simulink model "OptFahrzeug1"  (Simulink 5.1)
settings: Solver=ode5  StartTime=0.0  StopTime=max(sim_sample_time)  FixedStep=StepSize  RelTol=1e-3
values from neighbouring files (symbols this model uses):
  drive_acc =     [NoGenDoubleNEDC.mat]
  lm_alternator =     [NoGenDoubleNEDC.mat]
  PwpPt_Tq_EngGross = [0 0 0 1.18647349782e-14 1.38134887733e-14 1.57622425684e-14 1.77109963635e-14 1.96597501586e-14 2.16085039538e-14 2.35572577489e-14 2.5506011544e-14 2.74547653391e-14 ... (23602 elements, 23602x1)]    [NoGenDoubleNEDC.mat]    (also in newdoublecycle.m = [PwpPt_Tq_EngGross;PwpPt_Tq_EngGross])
  PwpPt_W_EngDn = [750 750 750 750 750 750 750 750 750 750 750 750 ... (23602 elements, 23602x1)]    [NoGenDoubleNEDC.mat]    (also in newdoublecycle.m = [PwpPt_W_EngDn;PwpPt_W_EngDn])
  sim_sample_time = [0 0.1 0.2 0.3 0.4 0.5 0.6 0.7 0.8 0.9 1 1.1 ... (23602 elements, 23602x1)]    [NoGenDoubleNEDC.mat]    (also in newdoublecycle.m = [sim_sample_time;sim_sample_time+max(sim_sample_time)+0.1])
  StromTraj = [36.79 ... (first row only)    [StromTrajDef.m]
  ZeitTraj = [0:0.1:-0.1+length(StromTraj)/10]'    [StromTrajDef.m]
settings Model: LastModifiedBy=meifert  ProdHWDeviceType=Microprocessor

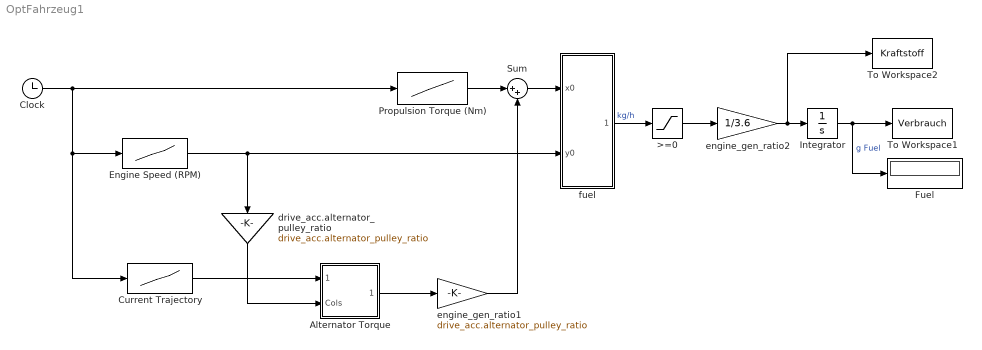
== system OptFahrzeug1 ==
  >=0 : Saturate  UpperLimit=inf  LowerLimit=0
  Alternator Torque : Subsystem  AncestorBlock=|  mask(Lookup Table (2-D)){x=lm_alternator.amp, y=lm_alternator.rpm, t=lm_alternator.loss}
      | simulink3/Functions
      | & Tables/Look-Up
      | Table (2-D)
      mask prompts: x "Row:"; y "Column:"; t "Table:"
      mask help: Performs 2-D linear interpolation of input values using the specified input/output table. Extrapolation is performed outside the table boundaries. The first dimension corresponds to the top (or left) input port.
      mask init:
      | [r,c]=size(t);
      | xt=reshape(x,prod(size(x)),1);
      | xi=xt(:,ones(1,c));
      | minx=min(x); maxx=max(x);
      | mint=min(min(t)); maxt=max(max(t));
      mask Display: plot(double(xi),double(t),double([minx maxx]),double([mint mint]),double([minx minx]),double([mint maxt]))
  Clock : Clock
      settings: Decimation=10
  Current Trajectory : Lookup  InputValues=ZeitTraj  OutputValues=StromTraj  SaturateOnIntegerOverflow=on
  Engine Speed (RPM) : Lookup  InputValues=sim_sample_time  OutputValues=PwpPt_W_EngDn  SaturateOnIntegerOverflow=on
  Fuel : Display
  Integrator : Integrator
  Propulsion Torque (Nm) : Lookup  InputValues=sim_sample_time  OutputValues=PwpPt_Tq_EngGross  SaturateOnIntegerOverflow=on
  Sum : Sum  Inputs=|++  SaturateOnIntegerOverflow=on  InputSameDT=on
  To Workspace1 : ToWorkspace  VariableName=Verbrauch  SampleTime=-1  SaveFormat=Array
  To Workspace2 : ToWorkspace  VariableName=Kraftstoff  SampleTime=-1  SaveFormat=Array
  drive_acc.alternator_pulley_ratio : Gain  Orientation=down  Gain=drive_acc.alternator_pulley_ratio  SaturateOnIntegerOverflow=on
  engine_gen_ratio1 : Gain  Gain=drive_acc.alternator_pulley_ratio  SaturateOnIntegerOverflow=on
  engine_gen_ratio2 : Gain  Gain=1/3.6  SaturateOnIntegerOverflow=on
  fuel : Subsystem  mask(2-D Table Lookup){@1=engine.tq, @2=engine.rpm, @3=engine.fuel}
      mask prompts: @1 "X Index"; @2 "Y Index"; @3 "Table"
      mask help:
      | Two Dimensional Table Lookup
      | The first input corresponds to X Index and the second input corresponds to the Y Index
      mask init:
      | xindex=@1; yindex=@2; table=@3; sftab2chk(xindex,yindex,table);
      mask Help: This block returns a linearly interpolated intersection from the table using the X index (which corresponds to the rows of the table) and the Y index (which corresponds to the columns of the table).  Extrapolation is used.
      mask Display: plot(-10,-10,110,110,[90,50,10],[90,40,30],[90,50,10],[50,26,20],[90,50,10],[22,13,10])
  wires:
  Integrator/1 -> To Workspace1/1, Fuel/1  "g Fuel"
  fuel/1(table out) -> >=0/1  "kg/h"
  >=0/1 -> engine_gen_ratio2/1
  Clock/1 -> Propulsion Torque (Nm)/1, Engine Speed (RPM)/1, Current Trajectory/1
  Engine Speed (RPM)/1 -> drive_acc.alternator_pulley_ratio/1, fuel/2(y0)
  Alternator Torque/1(Out1) -> engine_gen_ratio1/1
  Current Trajectory/1 -> Alternator Torque/1(Rows)
  engine_gen_ratio1/1 -> Sum/2
  Propulsion Torque (Nm)/1 -> Sum/1
  engine_gen_ratio2/1 -> Integrator/1, To Workspace2/1
  drive_acc.alternator_pulley_ratio/1 -> Alternator Torque/2(Cols)
  Sum/1 -> fuel/1(x0)

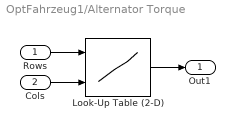
== system OptFahrzeug1/Alternator Torque ==
  Rows : Inport
  Cols : Inport  Port=2
  Look-Up Table (2-D) : Lookup2D  RowIndex=x  ColumnIndex=y  OutputValues=t  SaturateOnIntegerOverflow=on  InputSameDT=on
  Out1 : Outport
  wires:
  Rows/1 -> Look-Up Table (2-D)/1
  Cols/1 -> Look-Up Table (2-D)/2
  Look-Up Table (2-D)/1 -> Out1/1

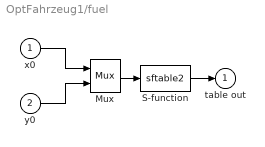
== system OptFahrzeug1/fuel ==
  x0 : Inport
  y0 : Inport  Port=2
  Mux : Mux  Inputs=2
  S-function : S-Function  FunctionName=sftable2  Parameters=xindex, yindex, table
  table out : Outport  InitialOutput=0
  wires:
  Mux/1 -> S-function/1
  x0/1 -> Mux/1
  S-function/1 -> table out/1
  y0/1 -> Mux/2
